simulink library "powerlib_models"  (Simulink 6.0)
settings: Solver=ode45  SolverMode=SingleTasking  StartTime=0.0  StopTime=10.0  RelTol=1e-3
values from neighbouring files (symbols this model uses):
  Ts = get(handles.edit1,'string')    [powergui.m]
undefined symbols (not defined in the file or in its folder): A, a0, a1, a2, a3, a4, a5, Ac, Amplitude, Amplitudes, B, BaseCurrent, BaseFlux, Bc, C, Capacitance, Cc, Columns, ConnectionType, Cs, ctrl, current, Current, damp, Dc, Dd, DiscIntNeverNeededParam, dref, dwo, exc, excAxis, F, Flux, fnom, Frequency, FreqVps, Gain1, gate, GH, GHd, GI, GId, GL, GLd, H, HarmonicGeneration, HT, hyd, I1_init, ib, ib2, Id1o, Inductance, InitialFlux, InitialSlope, io, Iq1o, isfinite, j, J ... (+138)
libraries: powerlib_models x32, powerlib_extras x4
(part 6 of 11)

== system powerlib_models/Continuous/GTO-IGBT Bridge/Vf  ==
  status_GTO : Inport  Port=1  LatchInput=off
  Switch : Switch  Threshold=0.5  InputSameDT=on
  Vf device : Constant  Value=Vf*ones(nb_switch,1)
  Vf diode : Constant  Value=-Vfd*ones(nb_switch,1)
  Vf : Outport  InitialOutput=[0]
  wires:
  status_GTO/1 -> Switch/2
  Switch/1 -> Vf/1
  Vf diode/1 -> Switch/3
  Vf device/1 -> Switch/1

== system powerlib_models/Continuous/HTG/PID ==
  error : Inport  Port=1  LatchInput=off
  Derivative : TransferFcn  Numerator=[ kd 0]  Denominator=[ td 1 ]
  Integral : Gain  Gain=ki  SaturateOnIntegerOverflow=on
  Integrator1 : Integrator  InitialCondition=go
  Proportional : Gain  Gain=kp  SaturateOnIntegerOverflow=on
  Sum : Sum  Inputs=+++  SaturateOnIntegerOverflow=on  InputSameDT=on
  Output : Outport  InitialOutput=0
  wires:
  Integrator1/1 -> Sum/2
  Integral/1 -> Integrator1/1
  error/1 -> Integral/1, Proportional/1, Derivative/1
  Sum/1 -> Output/1
  Derivative/1 -> Sum/3
  Proportional/1 -> Sum/1

== system powerlib_models/Continuous/HTG/servo-motor ==
  regulator's output : Inport  Port=1  LatchInput=off
  Sum4 : Sum  Inputs=+-  SaturateOnIntegerOverflow=on  InputSameDT=on
  position : Integrator  InitialCondition=go  LimitOutput=on  UpperSaturationLimit=gmax  LowerSaturationLimit=gmin
  servo- motor : TransferFcn  Numerator=[ka]  Denominator=[ta 1]
  speed limit : Saturate  UpperLimit=vgmax  LowerLimit=vgmin
  gate opening : Outport  InitialOutput=0
  wires:
  position/1 -> Sum4/2, gate opening/1
  speed limit/1 -> position/1
  servo- motor/1 -> speed limit/1
  Sum4/1 -> servo- motor/1
  regulator's output/1 -> Sum4/1

== system powerlib_models/Continuous/HTG/turbine ==
  dw : Inport  Port=1  LatchInput=off
  gate opening : Inport  Port=2  LatchInput=off
  Constant : Constant  Orientation=left
  Fcn : Fcn  Expr=(u(2)/u(1))^2
  Gain2 : Gain  Orientation=left  Gain=1/tw  SaturateOnIntegerOverflow=on
  Integrator : Integrator  Orientation=left  InitialCondition=po
  Mux : Mux  Inputs=2
  Product : Product  SaturateOnIntegerOverflow=on  InputSameDT=on
  Sum2 : Sum  Inputs=-+  SaturateOnIntegerOverflow=on  InputSameDT=on
  Sum3 : Sum  Orientation=left  Inputs=-+  SaturateOnIntegerOverflow=on  InputSameDT=on
  beta : Gain  Gain=beta  SaturateOnIntegerOverflow=on
  turbine gain : Gain  Gain=1/(gmax-gmin)  SaturateOnIntegerOverflow=on
  Pm : Outport  InitialOutput=0
  wires:
  turbine gain/1 -> Mux/1
  gate opening/1 -> turbine gain/1
  Integrator/1 -> Product/2, Mux/2
  Mux/1 -> Fcn/1
  Fcn/1 -> Sum2/2
  Constant/1 -> Sum3/2
  Product/1 -> Pm/1
  Sum3/1 -> Gain2/1
  Gain2/1 -> Integrator/1
  Sum2/1 -> Sum3/1, Product/1
  beta/1 -> Sum2/1
  dw/1 -> beta/1

== system powerlib_models/Continuous/MBPSS/Transfer function for detailed model (HF) ==
  On : Inport  Port=1  LatchInput=off
  "HFpos " : Inport  Port=2  LatchInput=off
  "HFneg " : Inport  Port=3  LatchInput=off
  Switch1 : Switch  Threshold=0.5  InputSameDT=on
  Switch2 : Switch  Threshold=0.5  InputSameDT=on
  Transfer functions for detailed stabilizer : Subsystem  TreatAsAtomicUnit=on
  Transfer functions for detailed stabilizer2 : Subsystem  TreatAsAtomicUnit=on
  HFpos : Outport
  HFneg : Outport  Port=2
  wires:
  Transfer functions for detailed stabilizer/1(Out1) -> Switch1/1
  "HFpos "/1 -> Transfer functions for detailed stabilizer/1(In1), Switch1/3
  Switch1/1 -> HFpos/1
  "HFneg "/1 -> Transfer functions for detailed stabilizer2/1(In1), Switch2/3
  Switch2/1 -> HFneg/1
  Transfer functions for detailed stabilizer2/1(Out1) -> Switch2/1
  On/1 -> Transfer functions for detailed stabilizer/Enable, Switch1/2, Switch2/2, Transfer functions for detailed stabilizer2/Enable

== system powerlib_models/Continuous/MBPSS/Transfer function for detailed model (IF) ==
  On : Inport  Port=1  LatchInput=off
  "IFpos " : Inport  Port=2  LatchInput=off
  "IFneg " : Inport  Port=3  LatchInput=off
  Switch1 : Switch  Threshold=0.5  InputSameDT=on
  Switch2 : Switch  Threshold=0.5  InputSameDT=on
  Transfer functions for detailed stabilizer : Subsystem  TreatAsAtomicUnit=on
  Transfer functions for detailed stabilizer2 : Subsystem  TreatAsAtomicUnit=on
  IFpos : Outport
  LFneg : Outport  Port=2
  wires:
  On/1 -> Transfer functions for detailed stabilizer2/Enable, Switch2/2, Switch1/2, Transfer functions for detailed stabilizer/Enable
  Transfer functions for detailed stabilizer2/1(Out1) -> Switch2/1
  Switch2/1 -> LFneg/1
  "IFneg "/1 -> Switch2/3, Transfer functions for detailed stabilizer2/1(In1)
  Switch1/1 -> IFpos/1
  "IFpos "/1 -> Switch1/3, Transfer functions for detailed stabilizer/1(In1)
  Transfer functions for detailed stabilizer/1(Out1) -> Switch1/1

== system powerlib_models/Continuous/MBPSS/Transfer function for detailed model (LF) ==
  On : Inport  Port=1  LatchInput=off
  "LFpos " : Inport  Port=2  LatchInput=off
  "LFneg " : Inport  Port=3  LatchInput=off
  Switch1 : Switch  Threshold=0.5  InputSameDT=on
  Switch2 : Switch  Threshold=0.5  InputSameDT=on
  Transfer functions for detailed stabilizer : Subsystem  TreatAsAtomicUnit=on
  Transfer functions for detailed stabilizer2 : Subsystem  TreatAsAtomicUnit=on
  LFpos : Outport
  LFneg : Outport  Port=2
  wires:
  Transfer functions for detailed stabilizer/1(Out1) -> Switch1/1
  "LFpos "/1 -> Transfer functions for detailed stabilizer/1(In1), Switch1/3
  Switch1/1 -> LFpos/1
  "LFneg "/1 -> Transfer functions for detailed stabilizer2/1(In1), Switch2/3
  Switch2/1 -> LFneg/1
  Transfer functions for detailed stabilizer2/1(Out1) -> Switch2/1
  On/1 -> Transfer functions for detailed stabilizer/Enable, Switch1/2, Switch2/2, Transfer functions for detailed stabilizer2/Enable

== system powerlib_models/Continuous/PM_synchronous_machine/abc2qd ==
  note: This subsystem converts Vab and Vbc to Vd,Vq. The sine and cosine com-
      | puted here are sent to the inverse transformation subsystem dq2abc.
  Vab,Vbc : Inport  Port=1  LatchInput=off
  the : Inport  Port=2  LatchInput=off
  Elementary Math : ElementaryMath
  Elementary Math1 : ElementaryMath  Operator=cos
  Fcn2 : Fcn  Expr=(u[4]*(2*u[1]+u[2]) + (sqrt3*u[2]*u[3])) * one_third
  Fcn3 : Fcn  Expr=(u[3]*(2*u[1]+u[2]) + (-sqrt3*u[2]*u[4])) * one_third
  Mux1 : Mux  Inputs=[ 2 2 ]
  Mux2 : Mux  Inputs=2
  Mux3 : Mux  Inputs=2
  s,c : Outport  InitialOutput=0
  vq,vd : Outport  Port=2  InitialOutput=0
  wires:
  the/1 -> Elementary Math1/1, Elementary Math/1
  Elementary Math1/1 -> Mux3/2
  Elementary Math/1 -> Mux3/1
  Vab,Vbc/1 -> Mux1/1
  Mux2/1 -> vq,vd/1
  Fcn3/1 -> Mux2/2
  Fcn2/1 -> Mux2/1
  Mux3/1 -> Mux1/2, s,c/1
  Mux1/1 -> Fcn3/1, Fcn2/1

== system powerlib_models/Continuous/PM_synchronous_machine/iq,id ==
  vq,vd : Inport  Port=1  LatchInput=off
  we : Inport  Port=2  LatchInput=off
  Demux : Demux  Outputs=2
  Mux : Mux  Inputs=2
  id : Subsystem
  iq : Subsystem
  iq,id : Outport  InitialOutput=0
  wires:
  Mux/1 -> iq,id/1
  vq,vd/1 -> Demux/1
  Demux/1 -> iq/1(vq)
  Demux/2 -> id/3(vd)
  iq/1(iq) -> id/1(iq), Mux/1
  we/1 -> id/2(we), iq/2(we)
  id/1(id) -> iq/3(id), Mux/2

== system powerlib_models/Continuous/PM_synchronous_machine/qd2abc ==
  s,c : Inport  Port=1  LatchInput=off
  iq,id : Inport  Port=2  LatchInput=off
  Fcn : Fcn  Expr=u[3]*u[2] + u[4]*u[1]
  Fcn1 : Fcn  Expr=(u[2]*(-u[3]-sqrt3*u[4]) + u[1]*(sqrt3*u[3]-u[4]))*0.5
  Mux : Mux  Inputs=[2,2]
  Mux2 : Mux  Inputs=3
  Sum : Sum  Orientation=down  Inputs=--  SaturateOnIntegerOverflow=on  InputSameDT=on
  is : Outport  InitialOutput=0
  wires:
  Mux2/1 -> is/1
  Fcn1/1 -> Sum/1, Mux2/2
  Fcn/1 -> Sum/2, Mux2/1
  Sum/1 -> Mux2/3
  iq,id/1 -> Mux/2
  s,c/1 -> Mux/1
  Mux/1 -> Fcn1/1, Fcn/1

== system powerlib_models/Continuous/PSS/Sensor ==
  In : Inport  Port=1  LatchInput=off
  State-Space : StateSpace  A=Ac  B=Bc  C=Cc  D=Dc  X0=x0c
  Out : Outport  InitialOutput=0
  wires:
  In/1 -> State-Space/1
  State-Space/1 -> Out/1

== system powerlib_models/Continuous/PSS/Wash-out ==
  In : Inport  Port=1  LatchInput=off
  State-Space : StateSpace  A=Ac  B=Bc  C=Cc  D=Dc  X0=x0c
  Out : Outport  InitialOutput=0
  wires:
  In/1 -> State-Space/1
  State-Space/1 -> Out/1

== system powerlib_models/Continuous/Three-Level Bridge/2-level GTO-IGBT Bridge  Logic (modified) ==
  note: Diode Logic :
      | 1) Diodes are blocked when complementary GTOs are switched on
  note: Note 3: See Sw3 logic
  v : Inport  Port=1  LatchInput=off
  g : Inport  Port=2  LatchInput=off
  Block12 : Inport  Port=3  LatchInput=off
  Trig12 : Inport  Port=4  LatchInput=off
  Data Type  Conversion2 : DataTypeConversion  OutDataTypeMode=double  SaturateOnIntegerOverflow=on  RndMeth=Zero
  Data Type  Conversion4 : DataTypeConversion  OutDataTypeMode=boolean  SaturateOnIntegerOverflow=on  RndMeth=Zero
  Demux1 : Demux  Outputs=[nb_arm nb_arm]
  Diode Logic : Subsystem
  GTO Logic : Subsystem
  G_D : Logic  Operator=OR
  G_D2 : Logic  Operator=NOT
  G_D3 : Logic  Operator=OR
  G_D4 : Logic  Operator=OR
  Gain : Gain  Orientation=up  Gain=-1  SaturateOnIntegerOverflow=on
  Gain1 : Gain  Gain=2  SaturateOnIntegerOverflow=on
  Memory : Memory
  Memory1 : Memory
  Note 3 : Logic
  Select_Block3 : Selector  Elements=Block3Elements  InputPortWidth=nb_switch
  Select_Vsw : Selector  Elements=VswElements  InputPortWidth=nb_arm*3
  "Vf " : Subsystem
  status : Outport
  Vf : Outport  Port=2
  Block3 : Outport  Port=3
  status_GTO : Outport  Port=4
  wires:
  Demux1/2 -> G_D3/2
  Demux1/1 -> G_D3/1
  Select_Block3/1 -> Demux1/1
  Select_Vsw/1 -> GTO Logic/1(Vak), Gain/1
  Trig12/1 -> G_D4/2
  Note 3/1 -> G_D4/1
  G_D4/1 -> G_D/1
  Memory/1 -> Vf/1
  Data Type  Conversion2/1 -> Memory1/1
  G_D/1 -> Data Type  Conversion2/1
  Memory1/1 -> status/1
  Data Type  Conversion4/1 -> GTO Logic/2(G)
  g/1 -> Data Type  Conversion4/1
  GTO Logic/1(status) -> status_GTO/1, "Vf "/1(status_GTO), Diode Logic/2(G), G_D/2
  "Vf "/1(Vf) -> Gain1/1
  v/1 -> Select_Vsw/1
  Gain/1 -> Diode Logic/1(Vak)
  Diode Logic/2(block) -> Select_Block3/1
  Diode Logic/1(status) -> Note 3/1
  Block12/1 -> G_D2/1
  G_D2/1 -> Note 3/2
  Gain1/1 -> Memory/1
  G_D3/1 -> Block3/1

== system powerlib_models/Continuous/Three-Level Bridge/Input ==
  note: This block is required when the "pulses" input is not connected
  In : Inport  Port=1  LatchInput=off
  Constant : Constant
  require : Logic  OutDataTypeMode=Specify via dialog  LogicDataType=float('double')
  Out : Outport
  wires:
  require/1 -> Out/1
  In/1 -> require/1
  Constant/1 -> require/2

== system powerlib_models/Continuous/Three-Level Bridge/SubSystem ==
  note: (or B or C)
  note: (or B or C)
  note: <======>
  note: |
      | |
      | |
      | |
      | |
      | [Sw2]
      | |
      | |
      | |
      | |
  note: |
      | |
      | |
      | |
      | |
      | [Sw1]
      | |
      | |
      | |
      | |
  note: + Vdc ------------
  note: ---------- A
  note: + Vdc --------------------------
  note: - Vdc--------------------------
  note: N ----------
  note: |
      | |
      | |
      | |
      | |
      | |
      | |
      | |
      | |
      | |
      | |
  note: ------------ A
  note: -----<-[D6]---------
  note: -------[D5]-->-------
  note: |
      | |
      | [Q4 - D4]
      | |
      | |
      | |
  note: |
      | |
      | [Q3 - D3]
      | |
      | |
  note: |
      | |
      | [Q2 - D2]
      | |
      | |
  note: |
      | |
      | |
      | [Q1 - D1]
      | |
      | |
  note: -[Sw3]-----
  note: N ----
  note: - Vdc ------------
  note: D5, D6 : Clamping diodes

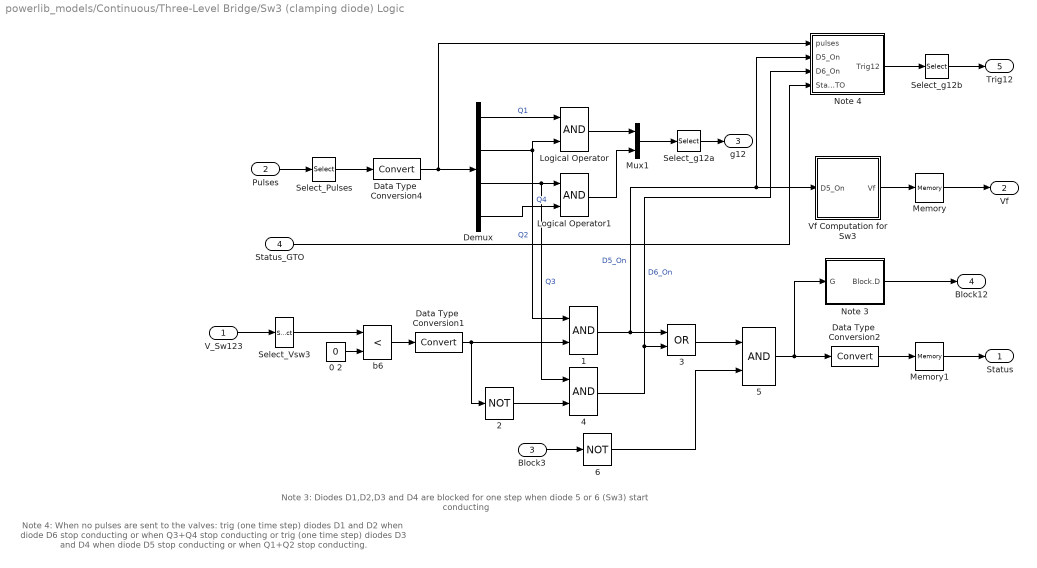
== system powerlib_models/Continuous/Three-Level Bridge/Sw3 (clamping diode) Logic ==
  note: Note 4: When no pulses are sent to the valves:
      | trig (one time step) diodes D1 and D2 when diode D6 stop conducting or when Q3+Q4 stop conducting
      | or trig (one time step) diodes D3 and D4 when diode D5 stop conducting or when Q1+Q2 stop conducting.
  note: Note 3: Diodes D1,D2,D3 and D4 are blocked for one step when diode 5 or 6 (Sw3) start conducting
  V_Sw123 : Inport  Port=1  LatchInput=off
  Pulses : Inport  Port=2  LatchInput=off
  Block3 : Inport  Port=3  LatchInput=off
  Status_GTO : Inport  Port=4  LatchInput=off
  0 2 : Constant  Value=0
  1 : Logic
  2 : Logic  Operator=NOT
  3 : Logic  Operator=OR
  4 : Logic
  5 : Logic
  6 : Logic  Operator=NOT
  Data Type  Conversion1 : DataTypeConversion  OutDataTypeMode=boolean  SaturateOnIntegerOverflow=on  RndMeth=Zero
  Data Type  Conversion2 : DataTypeConversion  OutDataTypeMode=double  SaturateOnIntegerOverflow=on  RndMeth=Zero
  Data Type  Conversion4 : DataTypeConversion  OutDataTypeMode=boolean  SaturateOnIntegerOverflow=on  RndMeth=Zero
  Demux : Demux  Outputs=[nb_arm nb_arm nb_arm nb_arm]
  Logical Operator : Logic
  Logical Operator1 : Logic
  Memory : Memory
  Memory1 : Memory
  Mux1 : Mux  Inputs=[nb_arm nb_arm]
  Note 3 : Subsystem
  Note 4 : Subsystem
  Select_Pulses : Selector  Elements=PulseElements  InputPortWidth=nb_arm*4
  Select_Vsw3 : Selector  Elements=Vsw3Elements  InputPortWidth=nb_arm*3
  Select_g12a : Selector  Elements=g12Elements  InputPortWidth=nb_arm*2
  Select_g12b : Selector  Elements=g12Elements  InputPortWidth=nb_arm*2
  Vf Computation for Sw3 : Subsystem
  b6 : RelationalOperator  Operator=<  InputSameDT=on
  Status : Outport
  Vf : Outport  Port=2
  g12 : Outport  Port=3
  Block12 : Outport  Port=4
  Trig12 : Outport  Port=5
  wires:
  Status_GTO/1 -> Note 4/4(Status_GTO)
  Select_Pulses/1 -> Data Type  Conversion4/1
  Note 4/1(Trig12) -> Select_g12b/1
  Data Type  Conversion2/1 -> Memory1/1
  6/1 -> 5/2
  3/1 -> 5/1
  1/1 -> Note 4/2(D5_On), Vf Computation for Sw3/1(D5_On), 3/1  "D5_On"
  4/1 -> Note 4/3(D6_On), 3/2  "D6_On"
  Data Type  Conversion1/1 -> 2/1, 1/2
  b6/1 -> Data Type  Conversion1/1
  Logical Operator1/1 -> Mux1/2
  Demux/4 -> Logical Operator1/2  "Q4"
  Demux/3 -> Logical Operator1/1, 4/1  "Q3"
  Demux/2 -> 1/1, Logical Operator/2  "Q2"
  Demux/1 -> Logical Operator/1  "Q1"
  Data Type  Conversion4/1 -> Note 4/1(pulses), Demux/1
  Memory/1 -> Vf/1
  Vf Computation for Sw3/1(Vf) -> Memory/1
  Mux1/1 -> Select_g12a/1
  Pulses/1 -> Select_Pulses/1
  0 2/1 -> b6/2
  V_Sw123/1 -> Select_Vsw3/1
  2/1 -> 4/2
  Memory1/1 -> Status/1
  Block3/1 -> 6/1
  Note 3/1(Block.D) -> Block12/1
  5/1 -> Data Type  Conversion2/1, Note 3/1(G)
  Select_Vsw3/1 -> b6/1
  Logical Operator/1 -> Mux1/1
  Select_g12a/1 -> g12/1
  Select_g12b/1 -> Trig12/1

== system powerlib_models/Continuous/asynchronous_machine/Mutual fluxes ==
  phiqr,phidr : Inport  Port=1  LatchInput=off
  phiqs,phids : Inport  Port=2  LatchInput=off
  1\Llr : Gain  Gain=1/Llr  SaturateOnIntegerOverflow=on
  1\Llr1 : Gain  Gain=Laq  SaturateOnIntegerOverflow=on
  1\Llr2 : Gain  Gain=Lad  SaturateOnIntegerOverflow=on
  1\Lls : Gain  Gain=1/Lls  SaturateOnIntegerOverflow=on
  Demux1 : Demux  Outputs=2
  Demux2 : Demux  Outputs=2
  Mux3 : Mux  Inputs=2
  Sum : Sum  Inputs=|++  SaturateOnIntegerOverflow=on  InputSameDT=on
  Sum1 : Sum  Inputs=++|  SaturateOnIntegerOverflow=on  InputSameDT=on
  phimq,phimd : Outport
  wires:
  Sum1/1 -> 1\Llr2/1
  phiqs,phids/1 -> 1\Lls/1
  phiqr,phidr/1 -> 1\Llr/1
  1\Llr/1 -> Demux1/1
  Demux1/1 -> Sum/1
  Sum/1 -> 1\Llr1/1
  1\Lls/1 -> Demux2/1
  Demux2/1 -> Sum/2
  Demux2/2 -> Sum1/2
  Demux1/2 -> Sum1/1
  1\Llr1/1 -> Mux3/1
  1\Llr2/1 -> Mux3/2
  Mux3/1 -> phimq,phimd/1

== system powerlib_models/Continuous/asynchronous_machine/Rotor ==
  vqr,vdr : Inport  Port=1  LatchInput=off
  w-wr : Inport  Port=2  LatchInput=off
  phimq,phimd : Inport  Port=3  LatchInput=off
  1\Llr : Gain  Gain=1/Llr  SaturateOnIntegerOverflow=on
  1\Llr1 : Gain  Gain=Rr  SaturateOnIntegerOverflow=on
  1\Llr2 : Gain  Gain=1/Llr  SaturateOnIntegerOverflow=on
  1\Llr3 : Gain  Gain=Rr  SaturateOnIntegerOverflow=on
  Demux : Demux  Outputs=2
  Demux1 : Demux  Outputs=2
  Mux2 : Mux  Inputs=2
  Mux3 : Mux  Inputs=2
  Product : Product  SaturateOnIntegerOverflow=on  InputSameDT=on
  Product1 : Product  Orientation=left  SaturateOnIntegerOverflow=on  InputSameDT=on
  Sum1 : Sum  Inputs=++-||  SaturateOnIntegerOverflow=on  InputSameDT=on
  Sum2 : Sum  Inputs=+--  SaturateOnIntegerOverflow=on  InputSameDT=on
  Sum3 : Sum  Inputs=+-|  SaturateOnIntegerOverflow=on  InputSameDT=on
  Sum4 : Sum  Inputs=-+|  SaturateOnIntegerOverflow=on  InputSameDT=on
  phidr : Integrator  InitialCondition=phirdo
  phiqr : Integrator  InitialCondition=phirqo
  web1 : Gain  Gain=web_psb  SaturateOnIntegerOverflow=on
  web_psb : Gain  Gain=web_psb  SaturateOnIntegerOverflow=on
  iqr,idr : Outport
  phiqr,phidr : Outport  Port=2
  wires:
  phimq,phimd/1 -> Demux1/1
  Demux1/1 -> Sum3/2
  Demux/1 -> Sum2/1
  Sum3/1 -> 1\Llr/1
  1\Llr1/1 -> Sum2/3
  1\Llr/1 -> 1\Llr1/1, Mux2/1  "iqr"
  Mux2/1 -> iqr,idr/1
  Demux1/2 -> Sum4/1
  Sum4/1 -> 1\Llr2/1
  1\Llr2/1 -> Mux2/2, 1\Llr3/1  "idr"
  1\Llr3/1 -> Sum1/3
  Demux/2 -> Sum1/2
  Product1/1 -> Sum1/1
  vqr,vdr/1 -> Demux/1
  phidr/1 -> Mux3/2, Product/1, Sum4/2
  Sum2/1 -> web_psb/1
  web_psb/1 -> phiqr/1
  Product/1 -> Sum2/2
  w-wr/1 -> Product1/1, Product/2
  Sum1/1 -> web1/1
  web1/1 -> phidr/1
  phiqr/1 -> Sum3/1, Product1/2, Mux3/1  "phiqr"
  Mux3/1 -> phiqr,phidr/1

== system powerlib_models/Continuous/asynchronous_machine/Stator ==
  phimq,phimd : Inport  Port=1  LatchInput=off
  vqs,vds : Inport  Port=2  LatchInput=off
  w : Inport  Port=3  LatchInput=off
  1\Llr : Gain  Gain=1/Lls  SaturateOnIntegerOverflow=on
  1\Llr1 : Gain  Gain=Rs  SaturateOnIntegerOverflow=on
  1\Llr2 : Gain  Gain=1/Lls  SaturateOnIntegerOverflow=on
  1\Llr3 : Gain  Gain=Rs  SaturateOnIntegerOverflow=on
  Demux : Demux  Outputs=2
  Demux1 : Demux  Outputs=2
  Mux2 : Mux  Inputs=2
  Mux3 : Mux  Inputs=2
  Mux4 : Mux  Inputs=2
  Product : Product  SaturateOnIntegerOverflow=on  InputSameDT=on
  Product1 : Product  SaturateOnIntegerOverflow=on  InputSameDT=on
  Sum1 : Sum  Inputs=++-||  SaturateOnIntegerOverflow=on  InputSameDT=on
  Sum2 : Sum  Inputs=--+  SaturateOnIntegerOverflow=on  InputSameDT=on
  Sum3 : Sum  Inputs=-+  SaturateOnIntegerOverflow=on  InputSameDT=on
  Sum4 : Sum  Inputs=+-|  SaturateOnIntegerOverflow=on  InputSameDT=on
  phids : Integrator  InitialCondition=phisdo
  phiqs : Integrator  InitialCondition=phisqo
  web1 : Gain  Gain=web_psb  SaturateOnIntegerOverflow=on
  web_psb : Gain  Gain=web_psb  SaturateOnIntegerOverflow=on
  phiqs,phids : Outport
  iqs,ids : Outport  Port=2
  phis,is : Outport  Port=3
  wires:
  Mux4/1 -> phis,is/1
  Mux3/1 -> Mux4/1, phiqs,phids/1
  Product1/1 -> Sum1/1
  Demux/2 -> Sum1/2
  phids/1 -> Mux3/2, Sum3/2, Product/2
  Sum1/1 -> web1/1
  web1/1 -> phids/1
  1\Llr3/1 -> Sum1/3
  1\Llr2/1 -> Mux2/2, 1\Llr3/1  "ids"
  Sum3/1 -> 1\Llr2/1
  Demux1/2 -> Sum3/1
  w/1 -> Product1/1, Product/1
  Mux2/1 -> Mux4/2, iqs,ids/1
  phiqs/1 -> Sum4/1, Product1/2, Mux3/1
  web_psb/1 -> phiqs/1
  Product/1 -> Sum2/2
  Demux/1 -> Sum2/3
  Sum2/1 -> web_psb/1
  vqs,vds/1 -> Demux/1
  1\Llr1/1 -> Sum2/1
  1\Llr/1 -> 1\Llr1/1, Mux2/1  "iqs"
  Sum4/1 -> 1\Llr/1
  Demux1/1 -> Sum4/2
  phimq,phimd/1 -> Demux1/1

== system powerlib_models/Continuous/asynchronous_machine/abc2qd ==
  v : Inport  Port=1  LatchInput=off
  sin,cos : Inport  Port=2  LatchInput=off
  1_Vb : Gain  Gain=1/Vb  SaturateOnIntegerOverflow=on
  Constant : Constant  Orientation=down  Value=ctrl==1
  Constant1 : Constant  Orientation=down  Value=ctrl==2
  Constant2 : Constant  Orientation=down  Value=ctrl==3
  Constant3 : Constant  Orientation=down  Value=ctrl
  Constant4 : Constant  Orientation=left  Value=ctrl
  Multiport Switch : MultiPortSwitch  Inputs=3  InputSameDT=on
  Multiport Switch1 : MultiPortSwitch  Inputs=3  InputSameDT=on
  Mux : Mux  Inputs=2
  Rotor reference frame : Subsystem  TreatAsAtomicUnit=on
      mask Display: disp('Rotor\nreference\nframe')
  Stationary reference frame : Subsystem  TreatAsAtomicUnit=on
      mask Display: disp('Stationary\nreference\nframe')
  Synchronous reference frame : Subsystem  TreatAsAtomicUnit=on
      mask Display: disp('Synchronous\nreference\nframe')
  transit : Subsystem
  vqr,vdr : Outport
  vqs,vds : Outport  Port=2
  wires:
  v/1 -> transit/1(vu)
  Constant/1 -> Rotor reference frame/Enable
  Constant1/1 -> Stationary reference frame/Enable
  Constant2/1 -> Synchronous reference frame/Enable
  Multiport Switch1/1 -> vqs,vds/1
  Rotor reference frame/1(vqr,vdr) -> Multiport Switch/2
  Stationary reference frame/1(vqr,vdr) -> Multiport Switch/3
  Synchronous reference frame/1(vqr,vdr) -> Multiport Switch/4
  Rotor reference frame/2(vqs,vds) -> Multiport Switch1/2
  Stationary reference frame/2(vqs,vds) -> Multiport Switch1/3
  Synchronous reference frame/2(vqs,vds) -> Multiport Switch1/4
  Multiport Switch/1 -> vqr,vdr/1
  sin,cos/1 -> Mux/2
  Mux/1 -> Rotor reference frame/1(In1), Stationary reference frame/1(In1), Synchronous reference frame/1(In1)
  1_Vb/1 -> Mux/1
  Constant3/1 -> Multiport Switch/1
  Constant4/1 -> Multiport Switch1/1
  transit/1(vr,vs) -> 1_Vb/1

== system powerlib_models/Continuous/asynchronous_machine/dq2abc ==
  sin,cos : Inport  Port=1  LatchInput=off
  iqr,idr : Inport  Port=2  LatchInput=off
  iqs,ids : Inport  Port=3  LatchInput=off
  Constant : Constant  Orientation=down  Value=ctrl==1
  Constant1 : Constant  Orientation=down  Value=ctrl==2
  Constant2 : Constant  Orientation=down  Value=ctrl==3
  Constant3 : Constant  Orientation=down  Value=ctrl
  Constant4 : Constant  Orientation=left  Value=ctrl
  Multiport Switch : MultiPortSwitch  Inputs=3  InputSameDT=on
  Multiport Switch1 : MultiPortSwitch  Inputs=3  InputSameDT=on
  Mux : Mux  Inputs=3
  Mux1 : Mux  Inputs=2
  Mux2 : Mux  Inputs=2
  Mux3 : Mux  Inputs=2
  Rotor reference frame : Subsystem  TreatAsAtomicUnit=on
      mask Display: disp('Rotor\nreference\nframe')
  Selector : Selector  Elements=elements2  InputPortWidth=4
  Stationary reference frame : Subsystem  TreatAsAtomicUnit=on
      mask Display: disp('Stationary\nreference\nframe')
  Sum2 : Sum  Inputs=-  SaturateOnIntegerOverflow=on  InputSameDT=on
  Sum3 : Sum  Inputs=-  SaturateOnIntegerOverflow=on  InputSameDT=on
  Synchronous reference frame : Subsystem  TreatAsAtomicUnit=on
      mask Display: disp('Synchronous\nreference\nframe')
  ib : Gain  Gain=ib  SaturateOnIntegerOverflow=on
  irab,isab : Outport
  irabc : Outport  Port=2
  isabc : Outport  Port=3
  wires:
  Constant/1 -> Rotor reference frame/Enable
  Constant1/1 -> Stationary reference frame/Enable
  Constant2/1 -> Synchronous reference frame/Enable
  Rotor reference frame/1(ira,irb) -> Multiport Switch/2
  Stationary reference frame/1(ira,irb) -> Multiport Switch/3
  Synchronous reference frame/1(ira,irb) -> Multiport Switch/4
  Stationary reference frame/2(isa,isb) -> Multiport Switch1/3
  Synchronous reference frame/2(isa,isb) -> Multiport Switch1/4
  Mux/1 -> Rotor reference frame/1(In1), Stationary reference frame/1(In1), Synchronous reference frame/1(In1)
  iqs,ids/1 -> Mux/2
  iqr,idr/1 -> Mux/1
  Multiport Switch/1 -> Mux2/1, Mux1/1, Sum2/1
  Mux2/1 -> irabc/1
  Multiport Switch1/1 -> Mux1/2, Sum3/1, Mux3/1
  Sum2/1 -> Mux2/2
  sin,cos/1 -> Mux/3
  Rotor reference frame/2(isa,isb) -> Multiport Switch1/2
  Mux1/1 -> ib/1
  Constant3/1 -> Multiport Switch/1
  Constant4/1 -> Multiport Switch1/1
  Sum3/1 -> Mux3/2
  Mux3/1 -> isabc/1
  ib/1 -> Selector/1
  Selector/1 -> irab,isab/1

== system powerlib_models/Continuous/asynchronous_machine/sin,cos ==
  thr,wr : Inport  Port=1  LatchInput=off
  Constant : Constant  Orientation=down  Value=ctrl<3
  Constant1 : Constant  Value=ctrl
  Constant2 : Constant  Value=0
  Constant3 : Constant  Orientation=down  Value=ctrl==3
  Constant4 : Constant  Value=ctrl
  Constant5 : Constant  Value=0
  Constant6 : Constant
  Gain : Gain  Gain=-1  SaturateOnIntegerOverflow=on
  Multiport Switch : MultiPortSwitch  Inputs=3  InputSameDT=on
  Multiport Switch1 : MultiPortSwitch  Inputs=3  InputSameDT=on
  Selector : Selector  InputPortWidth=2
  Selector1 : Selector  Elements=2  InputPortWidth=2
  Switch : Switch  Threshold=0.5  InputSameDT=on
  sin(beta),cos(beta),sin(th),cos(th) : Subsystem  TreatAsAtomicUnit=on
  sin(thr),cos(thr) : Subsystem  TreatAsAtomicUnit=on
  sin,cos : Outport
  w-wr : Outport  Port=2
  w : Outport  Port=3
  wires:
  Multiport Switch1/1 -> w/1
  Constant6/1 -> Multiport Switch1/4
  Constant5/1 -> Multiport Switch1/3
  Constant4/1 -> Multiport Switch1/1
  Selector1/1 -> Multiport Switch1/2, Gain/1
  Gain/1 -> Multiport Switch/3  "-wr"
  sin(beta),cos(beta),sin(th),cos(th)/1("sin(beta),cos(beta), sin(th),cos(th)") -> Switch/3
  sin(thr),cos(thr)/1(sin(thr),cos(thr)) -> Switch/1
  Multiport Switch/1 -> w-wr/1
  Constant2/1 -> Multiport Switch/2
  Constant1/1 -> Multiport Switch/1
  sin(beta),cos(beta),sin(th),cos(th)/2(we-wr) -> Multiport Switch/4
  Constant3/1 -> sin(beta),cos(beta),sin(th),cos(th)/Enable
  Switch/1 -> sin,cos/1
  Selector/1 -> sin(thr),cos(thr)/1(thr)
  thr,wr/1 -> Selector1/1, sin(beta),cos(beta),sin(th),cos(th)/1(thr,wr), Selector/1
  Constant/1 -> Switch/2, sin(thr),cos(thr)/Enable

== system powerlib_models/Continuous/breaker/Break Algebraic Loop ==
  In1 : Inport  Port=1  LatchInput=off
  0 2 : Constant  Value=0.001
  Data Type  Conversion : DataTypeConversion  OutDataTypeMode=double  SaturateOnIntegerOverflow=on  RndMeth=Zero
  Data Type  Conversion1 : DataTypeConversion  OutDataTypeMode=double  SaturateOnIntegerOverflow=on  RndMeth=Zero
  Integrator : Integrator  InitialCondition=0.00101*(istate&1)  LimitOutput=on  UpperSaturationLimit=0.00101
  R_device : Gain  Gain=1e7  SaturateOnIntegerOverflow=on
  Relational Operator1 : RelationalOperator  Operator=>  InputSameDT=on
  Vak-Vf-Ron*Iak : Sum  Inputs=+-  SaturateOnIntegerOverflow=on  InputSameDT=on
  Out1 : Outport
  wires:
  Data Type  Conversion/1 -> Out1/1
  In1/1 -> Data Type  Conversion1/1
  Data Type  Conversion1/1 -> Vak-Vf-Ron*Iak/1
  R_device/1 -> Integrator/1
  Vak-Vf-Ron*Iak/1 -> R_device/1
  Integrator/1 -> Vak-Vf-Ron*Iak/2, Relational Operator1/1
  0 2/1 -> Relational Operator1/2
  Relational Operator1/1 -> Data Type  Conversion/1

== system powerlib_models/Continuous/detailed_thyristor (logical)/Break Alg. Loop ==
  In1 : Inport  Port=1  LatchInput=off
  0 2 : Constant  Value=0.001
  Data Type  Conversion : DataTypeConversion  OutDataTypeMode=double  SaturateOnIntegerOverflow=on  RndMeth=Zero
  Data Type  Conversion1 : DataTypeConversion  OutDataTypeMode=double  SaturateOnIntegerOverflow=on  RndMeth=Zero
  Integrator : Integrator  LimitOutput=on  UpperSaturationLimit=0.00101
  R_device : Gain  Gain=1e7  SaturateOnIntegerOverflow=on
  Relational Operator1 : RelationalOperator  Operator=>  InputSameDT=on
  Vak-Vf-Ron*Iak : Sum  Inputs=+-  SaturateOnIntegerOverflow=on  InputSameDT=on
  Out1 : Outport
  wires:
  Relational Operator1/1 -> Data Type  Conversion/1
  0 2/1 -> Relational Operator1/2
  Integrator/1 -> Relational Operator1/1, Vak-Vf-Ron*Iak/2
  Vak-Vf-Ron*Iak/1 -> R_device/1
  R_device/1 -> Integrator/1
  Data Type  Conversion1/1 -> Vak-Vf-Ron*Iak/1
  In1/1 -> Data Type  Conversion1/1
  Data Type  Conversion/1 -> Out1/1

== system powerlib_models/Continuous/diode (logical)/Break Alg. Loop ==
  In1 : Inport  Port=1  LatchInput=off
  0 2 : Constant  Value=0.001
  Data Type  Conversion : DataTypeConversion  OutDataTypeMode=double  SaturateOnIntegerOverflow=on  RndMeth=Zero
  Data Type  Conversion1 : DataTypeConversion  OutDataTypeMode=double  SaturateOnIntegerOverflow=on  RndMeth=Zero
  Integrator : Integrator  LimitOutput=on  UpperSaturationLimit=0.00101
  R_device : Gain  Gain=1e7  SaturateOnIntegerOverflow=on
  Relational Operator1 : RelationalOperator  Operator=>  InputSameDT=on
  Vak-Vf-Ron*Iak : Sum  Inputs=+-  SaturateOnIntegerOverflow=on  InputSameDT=on
  Out1 : Outport
  wires:
  Relational Operator1/1 -> Data Type  Conversion/1
  0 2/1 -> Relational Operator1/2
  Integrator/1 -> Relational Operator1/1, Vak-Vf-Ron*Iak/2
  Vak-Vf-Ron*Iak/1 -> R_device/1
  R_device/1 -> Integrator/1
  Data Type  Conversion1/1 -> Vak-Vf-Ron*Iak/1
  In1/1 -> Data Type  Conversion1/1
  Data Type  Conversion/1 -> Out1/1

== system powerlib_models/Continuous/hysteresis_transformer/Hysteresis ( always SI ) ==
  In1 : Inport  Port=1  LatchInput=off
  Hysteresis main loop + Saturation (Lower Part) : Lookup  DialogController=Simulink.DDGSource  InputValues=LowerFlux  OutputValues=Current  SaturateOnIntegerOverflow=on
  Hysteresis main loop + Saturation. (Upper Part) : Lookup  DialogController=Simulink.DDGSource  InputValues=UpperFlux  OutputValues=Current  SaturateOnIntegerOverflow=on
  Memory : Memory
  SI conversion : Gain  Gain=CurrentBase  SaturateOnIntegerOverflow=on
  Selector : Selector  Elements=2  InputPortWidth=2
  Selector1 : Selector  InputPortWidth=2
  Sfunction : S-Function  FunctionName=sfun_hysteresis  Parameters=sfun_InitialFlux,HT,TransfoNumber,-1,Tolerances,InitialSlope
  Sign : Signum
  Sum : Sum  Inputs=|+-  SaturateOnIntegerOverflow=on  InputSameDT=on
  Switch1 : Switch  InputSameDT=on
  Switch2 : Switch  Threshold=1.5  InputSameDT=on
  pu conversion : Gain  Gain=1/FluxBase  SaturateOnIntegerOverflow=on
  Out1 : Outport
  wires:
  Sum/1 -> Sign/1
  SI conversion/1 -> Switch2/1  "internal loops"
  Selector1/1 -> SI conversion/1
  Selector/1 -> Switch2/2  "Tr"
  Switch1/1 -> Switch2/3
  Switch2/1 -> Out1/1
  Sfunction/1 -> Selector1/1, Selector/1
  pu conversion/1 -> Sfunction/1
  Sign/1 -> Switch1/2
  Memory/1 -> Sum/2
  Hysteresis main loop + Saturation. (Upper Part)/1 -> Switch1/3
  In1/1 -> Sum/1, Memory/1, Hysteresis main loop + Saturation. (Upper Part)/1, Hysteresis main loop + Saturation (Lower Part)/1, pu conversion/1
  Hysteresis main loop + Saturation (Lower Part)/1 -> Switch1/1

== system powerlib_models/Continuous/simplified_sync_mach/Subsystem ==
  i : Inport  Port=1  LatchInput=off
  v : Inport  Port=2  LatchInput=off
  e : Inport  Port=3  LatchInput=off
  theta : Inport  Port=4  LatchInput=off
  wm : Inport  Port=5  LatchInput=off
  Pe : Inport  Port=6  LatchInput=off
  Gain : Gain  Gain=[ ib2*ones(3,1); Vb3*ones(6,1); 1; Nb; Pb ]  SaturateOnIntegerOverflow=on
  Mux : Mux  Inputs=[ 3 3 3 1 1 1 ]
  * : Outport  InitialOutput=0
  wires:
  Gain/1 -> */1
  Mux/1 -> Gain/1
  Pe/1 -> Mux/6
  wm/1 -> Mux/5
  theta/1 -> Mux/4
  e/1 -> Mux/3
  v/1 -> Mux/2
  i/1 -> Mux/1

== system powerlib_models/Continuous/simplified_sync_mach/Vt ==
  note: This subsystem either converts 2 line-to-line voltages to 3 line-to-neutral voltages (internal neutral)
      | and computes floating neutral voltage or directly passes Van,Vbn,Vcn if 4-wire connection.
  V : Inport  Port=1  LatchInput=off
  1_Vb : Gain  Gain=1/Vb  SaturateOnIntegerOverflow=on
  Constant : Constant  Orientation=left  Value=ConnectionType
  Constant1 : Constant  Value=0
  Constant2 : Constant  Value=0
  Data Type  Conversion1 : DataTypeConversion  Orientation=left  OutDataTypeMode=boolean  SaturateOnIntegerOverflow=on  RndMeth=Zero
  Data Type  Conversion2 : DataTypeConversion  OutDataTypeMode=double  SaturateOnIntegerOverflow=on  RndMeth=Zero
  Fcn : Fcn  Expr=u[1]
  Fcn1 : Fcn  Expr=u[2]
  Fcn2 : Fcn  Expr=u[3]
  Gain : Gain  Gain=1/3  SaturateOnIntegerOverflow=on
  LL2LN : Subsystem  TreatAsAtomicUnit=on
  Logical Operator : Logic  Operator=NOT
  Mux : Mux  Inputs=2
  Mux1 : Mux  Inputs=3
  Product : Product  SaturateOnIntegerOverflow=on  InputSameDT=on
  Sum : Sum  Inputs=+  SaturateOnIntegerOverflow=on  InputSameDT=on
  Sum1 : Sum  Inputs=|++  SaturateOnIntegerOverflow=on  InputSameDT=on
  Switch2 : Switch  Threshold=0.5  InputSameDT=on
  Vn : Outport  InitialOutput=0
  Vabc : Outport  Port=2  InitialOutput=0
  wires:
  Data Type  Conversion2/1 -> Product/1
  Logical Operator/1 -> Data Type  Conversion2/1
  Data Type  Conversion1/1 -> Logical Operator/1
  Constant/1 -> Data Type  Conversion1/1, LL2LN/Enable, Switch2/2
  Sum/1 -> Gain/1
  Gain/1 -> Switch2/1
  Constant2/1 -> Switch2/3
  Switch2/1 -> Vn/1
  LL2LN/1(Out1) -> Sum/1, Sum1/1
  Sum1/1 -> Vabc/1
  Constant1/1 -> Mux/2
  Mux/1 -> Fcn/1, Fcn1/1, Fcn2/1
  Fcn/1 -> Mux1/1
  Fcn1/1 -> Mux1/2
  Fcn2/1 -> Mux1/3
  Mux1/1 -> Product/2
  Product/1 -> Sum1/2
  V/1 -> 1_Vb/1
  1_Vb/1 -> LL2LN/1(In1), Mux/1

== system powerlib_models/Continuous/simplified_sync_mach/Z ==
  note: This subsystem models the internal impedance of
      | the machine, which consists of  a series RL circuit.
  e : Inport  Port=1  LatchInput=off
  v : Inport  Port=2  LatchInput=off
  1/L : Gain  Gain=web_psb/L  SaturateOnIntegerOverflow=on
  Integrator3 : Integrator  InitialCondition=io
  R : Gain  Orientation=left  Gain=R  SaturateOnIntegerOverflow=on
  Sum5 : Sum  Inputs=-+-  SaturateOnIntegerOverflow=on  InputSameDT=on
  i : Outport  InitialOutput=0
  wires:
  Integrator3/1 -> i/1, R/1
  1/L/1 -> Integrator3/1
  v/1 -> Sum5/3
  Sum5/1 -> 1/L/1
  R/1 -> Sum5/1
  e/1 -> Sum5/2

== system powerlib_models/Continuous/simplified_sync_mach/gen ==
  note: This subsystem generates the 3 line-to-neutral voltages inside the machine.
  theta : Inport  Port=1  LatchInput=off
  E : Inport  Port=2  LatchInput=off
  Vn : Inport  Port=3  LatchInput=off
  1_Vb2 : Gain  Gain=1/Vb2  SaturateOnIntegerOverflow=on
  Mux : Mux  Inputs=3
  Product : Product  SaturateOnIntegerOverflow=on  InputSameDT=on
  Sum : Sum  Inputs=|++  SaturateOnIntegerOverflow=on  InputSameDT=on
  Sum1 : Sum  Orientation=down  Inputs=--  SaturateOnIntegerOverflow=on  InputSameDT=on
  rem(wt,2pi) : Fcn  Expr=rem(u[1],2*pi)
  sin(a) : Fcn  Expr=sin(u)
  sin(b) : Fcn  Expr=sin(u-pi23)
  e : Outport  InitialOutput=0
  wires:
  rem(wt,2pi)/1 -> sin(a)/1, sin(b)/1
  theta/1 -> rem(wt,2pi)/1
  sin(a)/1 -> Sum1/2, Mux/1
  Sum1/1 -> Mux/3
  sin(b)/1 -> Sum1/1, Mux/2
  E/1 -> 1_Vb2/1
  1_Vb2/1 -> Product/2
  Vn/1 -> Sum/2
  Mux/1 -> Product/1
  Product/1 -> Sum/1
  Sum/1 -> e/1

== system powerlib_models/Continuous/simplified_sync_mach/wattmeter ==
  note: This subsystem computes the total electrical
      | power delivered or absorbed by the machine.
  i : Inport  Port=1  LatchInput=off
  v : Inport  Port=2  LatchInput=off
  2_3 : Gain  Gain=2/3  SaturateOnIntegerOverflow=on
  Product : Product  SaturateOnIntegerOverflow=on  InputSameDT=on
  Sum : Sum  Inputs=+  SaturateOnIntegerOverflow=on  InputSameDT=on
  Pe : Outport  InitialOutput=0
  wires:
  Product/1 -> Sum/1
  i/1 -> Product/1
  v/1 -> Product/2
  Sum/1 -> 2_3/1
  2_3/1 -> Pe/1

== system powerlib_models/Continuous/synchronous_machine/Delta angle ==
  Vq : Inport  Port=1  PortDimensions=1  LatchInput=off
  Vd : Inport  Port=2  PortDimensions=1  LatchInput=off
  Cartesian to Polar : Subsystem
      mask Type: Cart2Polar
      mask Description:
      | Transformation from cartesian to polar coordinates.
      | [x, y] -> [r, theta]
      | 
      | r = sqrt(x^2 + y^2);
      | theta = atan(y/x);
      mask Help: Unmask this block for more help.
      mask Display: plot(0,0,100,100,[24,20,15,20,20],[85,95,85,95,20],[80,20,95,85,95,85],[70,20,20,15,20,24],[56,56,55,52,50,46],[20,26,31,35,38,42])
  Radians to Degrees : Subsystem
      mask Type: RadiansToDegrees
      mask Description:
      | Conversion from Radians to Degrees.
      | 
      | D=180/pi*R
      mask Help: This block converts from Radians to Degrees.
      mask Display: disp('R2D')
  Terminator2 : Terminator
  delta : Outport
  wires:
  Cartesian to Polar/2(theta) -> Radians to Degrees/1(Radians in)
  Cartesian to Polar/1(r) -> Terminator2/1
  Vq/1 -> Cartesian to Polar/1(x)
  Radians to Degrees/1(Degrees out) -> delta/1  "delta"
  Vd/1 -> Cartesian to Polar/2(y)

== system powerlib_models/Continuous/synchronous_machine/PQ ==
  note: PQ Measurement:
  note: Q = Vq*Id-Vd*Iq
  note: P = Vd*Id + Vq*Iq
  Vq : Inport  Port=1  PortDimensions=1  LatchInput=off
  Vd : Inport  Port=2  PortDimensions=1  LatchInput=off
  Iq : Inport  Port=3  PortDimensions=2  LatchInput=off
  Demux1 : Demux  Outputs=[1,1]
  Gain : Gain  Gain=Gain1  SaturateOnIntegerOverflow=on
  Gain1 : Gain  Gain=Gain1  SaturateOnIntegerOverflow=on
  Product{2..5} (4 alike) : Product  SaturateOnIntegerOverflow=on  InputSameDT=on
  Sum : Sum  SaturateOnIntegerOverflow=on  InputSameDT=on
  Sum1 : Sum  Inputs=+-  SaturateOnIntegerOverflow=on  InputSameDT=on
  Peo : Outport
  Qeo : Outport  Port=2
  wires:
  Demux1/2 -> Product4/2, Product3/2
  Vq/1 -> Product4/1, Product2/1
  Vd/1 -> Product5/1, Product3/1
  Sum1/1 -> Gain1/1  "Qeo"
  Sum/1 -> Gain/1  "Peo"
  Product5/1 -> Sum1/2
  Product4/1 -> Sum1/1
  Product3/1 -> Sum/2
  Product2/1 -> Sum/1
  Gain/1 -> Peo/1
  Gain1/1 -> Qeo/1
  Iq/1 -> Demux1/1
  Demux1/1 -> Product2/2, Product5/2

== system powerlib_models/Continuous/synchronous_machine/Subsystem ==
  Vf : Inport  Port=1  PortDimensions=1  LatchInput=off
  Constant : Constant  Value=excAxis
  Ground2 : Ground
  Switch : Switch  Threshold=1.5  InputSameDT=on
  Switch1 : Switch  Threshold=1.5  InputSameDT=on
  Vkq1 : Outport
  Vfd : Outport  Port=2
  wires:
  Ground2/1 -> Switch1/1, Switch/3
  Vf/1 -> Switch1/3, Switch/1
  Constant/1 -> Switch/2, Switch1/2
  Switch1/1 -> Vfd/1
  Switch/1 -> Vkq1/1

== system powerlib_models/Continuous/synchronous_machine/abc2qd ==
  note: This subsystem converts Vab and Vbc to Vd,Vq. The sine and cosine com-
      | puted here are sent to the inverse transformation subsystem qd/abc.
  v : Inport  Port=1  PortDimensions=2  LatchInput=off
  theta : Inport  Port=2  PortDimensions=1  LatchInput=off
  1_Vb : Gain  Gain=1/Vb  SaturateOnIntegerOverflow=on
  Elementary Math : ElementaryMath
  Elementary Math1 : ElementaryMath  Operator=cos
  Fcn2 : Fcn  Expr=(u[4]*(2*u[1]+u[2]) + (sqrt3*u[2]*u[3])) * one_third
  Fcn3 : Fcn  Expr=(u[3]*(2*u[1]+u[2]) + (-sqrt3*u[2]*u[4])) * one_third
  Mux1 : Mux  Inputs=[ 2 2 ]
  Mux3 : Mux  Inputs=2
  cos,sin : Outport  InitialOutput=0
  vq : Outport  Port=2  InitialOutput=0
  vd : Outport  Port=3  InitialOutput=0
  wires:
  1_Vb/1 -> Mux1/1
  v/1 -> 1_Vb/1
  Mux1/1 -> Fcn2/1, Fcn3/1
  Mux3/1 -> Mux1/2, cos,sin/1
  theta/1 -> Elementary Math/1, Elementary Math1/1
  Elementary Math/1 -> Mux3/1
  Elementary Math1/1 -> Mux3/2
  Fcn2/1 -> vq/1  "vq"
  Fcn3/1 -> vd/1  "vd"

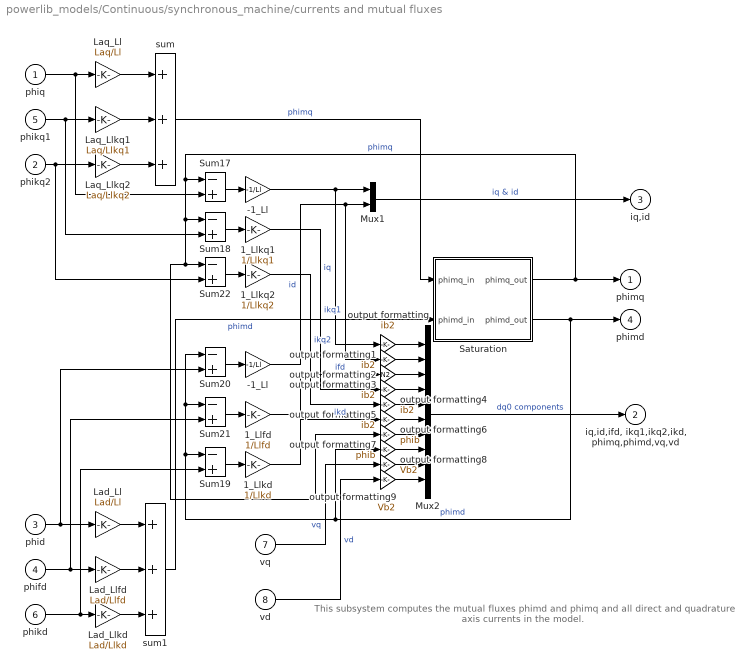
== system powerlib_models/Continuous/synchronous_machine/currents and mutual fluxes ==
  note: This subsystem computes the mutual fluxes phimd
      | and phimq and all direct and quadrature axis
      | currents in the model.
  phiq : Inport  Port=1  PortDimensions=1  LatchInput=off
  phikq2 : Inport  Port=2  PortDimensions=1  LatchInput=off
  phid : Inport  Port=3  PortDimensions=1  LatchInput=off
  phifd : Inport  Port=4  PortDimensions=1  LatchInput=off
  phikq1 : Inport  Port=5  PortDimensions=1  LatchInput=off
  phikd : Inport  Port=6  PortDimensions=1  LatchInput=off
  vq : Inport  Port=7  PortDimensions=1  LatchInput=off
  vd : Inport  Port=8  PortDimensions=1  LatchInput=off
  -1_Ll : Gain  Gain=-1/Ll  SaturateOnIntegerOverflow=on
  "-1_Ll " : Gain  Gain=-1/Ll  SaturateOnIntegerOverflow=on
  1_Llfd : Gain  Gain=1/Llfd  SaturateOnIntegerOverflow=on
  1_Llkd : Gain  Gain=1/Llkd  SaturateOnIntegerOverflow=on
  1_Llkq1 : Gain  Gain=1/Llkq1  SaturateOnIntegerOverflow=on
  1_Llkq2 : Gain  Gain=1/Llkq2  SaturateOnIntegerOverflow=on
  Lad_Ll : Gain  Gain=Lad/Ll  SaturateOnIntegerOverflow=on
  Lad_Llfd : Gain  Gain=Lad/Llfd  SaturateOnIntegerOverflow=on
  Lad_Llkd : Gain  Gain=Lad/Llkd  SaturateOnIntegerOverflow=on
  Laq_Ll : Gain  Gain=Laq/Ll  SaturateOnIntegerOverflow=on
  Laq_Llkq1 : Gain  Gain=Laq/Llkq1  SaturateOnIntegerOverflow=on
  Laq_Llkq2 : Gain  Gain=Laq/Llkq2  SaturateOnIntegerOverflow=on
  Mux1 : Mux  Inputs=2
  Mux2 : Mux  Inputs=[1,1,1,1,1,1,1,1,1,1]
  Saturation : Subsystem
  Sum{17..22} (6 alike) : Sum  Inputs=-+  SaturateOnIntegerOverflow=on  InputSameDT=on
  output formatting{,1,3..5} (5 alike) : Gain  Gain=ib2  SaturateOnIntegerOverflow=on
  output formatting2 : Gain  Gain=N2  SaturateOnIntegerOverflow=on
  output formatting6 : Gain  Gain=phib  SaturateOnIntegerOverflow=on
  output formatting7 : Gain  Gain=phib  SaturateOnIntegerOverflow=on
  output formatting8 : Gain  Gain=Vb2  SaturateOnIntegerOverflow=on
  output formatting9 : Gain  Gain=Vb2  SaturateOnIntegerOverflow=on
  sum : Sum  Inputs=+++  SaturateOnIntegerOverflow=on  InputSameDT=on
  sum1 : Sum  Inputs=+++  SaturateOnIntegerOverflow=on  InputSameDT=on
  phimq : Outport  InitialOutput=0
  "iq,id,ifd, ikq1,ikq2,ikd, phimq,phimd,vq,vd" : Outport  Port=2  InitialOutput=0
  iq,id : Outport  Port=3  InitialOutput=0
  phimd : Outport  Port=4  InitialOutput=0
  wires:
  Saturation/2(phimd_out) -> Sum19/1, Sum21/1, Sum20/1, output formatting7/1, phimd/1  "phimd"
  Saturation/1(phimq_out) -> Sum17/1, Sum22/1, output formatting6/1, Sum18/1, phimq/1  "phimq"
  sum1/1 -> Saturation/2(phimd_in)  "phimd"
  sum/1 -> Saturation/1(phimq_in)  "phimq"
  1_Llkq2/1 -> output formatting4/1  "ikq2"
  1_Llkq1/1 -> output formatting3/1  "ikq1"
  Sum20/1 -> "-1_Ll "/1
  "-1_Ll "/1 -> Mux1/2, output formatting1/1  "id"
  Sum21/1 -> 1_Llfd/1
  Sum19/1 -> 1_Llkd/1
  1_Llfd/1 -> output formatting2/1  "ifd"
  1_Llkd/1 -> output formatting5/1  "ikd"
  Sum18/1 -> 1_Llkq1/1
  Sum17/1 -> -1_Ll/1
  Sum22/1 -> 1_Llkq2/1
  -1_Ll/1 -> Mux1/1, output formatting/1  "iq"
  Mux1/1 -> iq,id/1  "iq & id"
  Lad_Llkd/1 -> sum1/3
  Lad_Llfd/1 -> sum1/2
  Lad_Ll/1 -> sum1/1
  phifd/1 -> Lad_Llfd/1, Sum21/2
  phid/1 -> Sum20/2, Lad_Ll/1
  phikd/1 -> Lad_Llkd/1, Sum19/2
  phiq/1 -> Laq_Ll/1, Sum17/2
  Laq_Ll/1 -> sum/1
  Laq_Llkq2/1 -> sum/3
  Laq_Llkq1/1 -> sum/2
  phikq2/1 -> Laq_Llkq2/1, Sum22/2
  phikq1/1 -> Laq_Llkq1/1, Sum18/2
  vq/1 -> output formatting8/1  "vq"
  vd/1 -> output formatting9/1  "vd"
  Mux2/1 -> "iq,id,ifd, ikq1,ikq2,ikd, phimq,phimd,vq,vd"/1  "dq0 components"
  output formatting/1 -> Mux2/1
  output formatting1/1 -> Mux2/2
  output formatting2/1 -> Mux2/3
  output formatting3/1 -> Mux2/4
  output formatting4/1 -> Mux2/5
  output formatting5/1 -> Mux2/6
  output formatting6/1 -> Mux2/7
  output formatting7/1 -> Mux2/8
  output formatting8/1 -> Mux2/9
  output formatting9/1 -> Mux2/10

== system powerlib_models/Continuous/synchronous_machine/phid ==
  note: This subsystem computes the direct axis flux phid.
  w : Inport  Port=1  PortDimensions=1  LatchInput=off
  phiq : Inport  Port=2  PortDimensions=1  LatchInput=off
  vd : Inport  Port=3  PortDimensions=1  LatchInput=off
  phimd : Inport  Port=4  PortDimensions=1  LatchInput=off
  Product1 : Product  SaturateOnIntegerOverflow=on  InputSameDT=on
  Rs_Ll : Gain  Gain=Rs/Ll  SaturateOnIntegerOverflow=on
  Sum2 : Sum  Inputs=+++  SaturateOnIntegerOverflow=on  InputSameDT=on
  Sum9 : Sum  Inputs=+-  SaturateOnIntegerOverflow=on  InputSameDT=on
  int : Integrator  InitialCondition=phido
  web_psb : Gain  Gain=web_psb  SaturateOnIntegerOverflow=on
  phid : Outport  InitialOutput=0
  wires:
  phimd/1 -> Sum9/1
  vd/1 -> Sum2/2
  phiq/1 -> Product1/2
  w/1 -> Product1/1
  Product1/1 -> Sum2/1
  Sum9/1 -> Rs_Ll/1
  Rs_Ll/1 -> Sum2/3
  Sum2/1 -> web_psb/1
  web_psb/1 -> int/1
  int/1 -> phid/1, Sum9/2

== system powerlib_models/Continuous/synchronous_machine/phifd ==
  note: This subsystem computes the field flux phifd.
  vfd : Inport  Port=1  PortDimensions=1  LatchInput=off
  phimd : Inport  Port=2  PortDimensions=1  LatchInput=off
  N : Gain  Gain=N  SaturateOnIntegerOverflow=on
  Rf_Llfd : Gain  Gain=Rf/Llfd  SaturateOnIntegerOverflow=on
  Sum10 : Sum  Inputs=+-  SaturateOnIntegerOverflow=on  InputSameDT=on
  Sum3 : Sum  SaturateOnIntegerOverflow=on  InputSameDT=on
  int : Integrator  InitialCondition=phifdo
  web_psb : Gain  Gain=web_psb  SaturateOnIntegerOverflow=on
  phifd : Outport  InitialOutput=0
  wires:
  N/1 -> Sum3/1
  vfd/1 -> N/1
  Rf_Llfd/1 -> Sum3/2
  Sum10/1 -> Rf_Llfd/1
  phimd/1 -> Sum10/1
  web_psb/1 -> int/1
  int/1 -> phifd/1, Sum10/2
  Sum3/1 -> web_psb/1

== system powerlib_models/Continuous/synchronous_machine/phikd ==
  note: This subsystem computes the direct axis damper flux phikd.
  phimd : Inport  Port=1  PortDimensions=1  LatchInput=off
  vkd : Inport  Port=2  PortDimensions=1  LatchInput=off
  Rkd_Llkd : Gain  Gain=Rkd/Llkd  SaturateOnIntegerOverflow=on
  Sum11 : Sum  Inputs=-+  SaturateOnIntegerOverflow=on  InputSameDT=on
  Sum4 : Sum  SaturateOnIntegerOverflow=on  InputSameDT=on
  int : Integrator  InitialCondition=phikdo
  web_psb : Gain  Gain=web_psb  SaturateOnIntegerOverflow=on
  phikd : Outport  InitialOutput=0
  wires:
  Rkd_Llkd/1 -> Sum4/1
  Sum11/1 -> Rkd_Llkd/1
  phimd/1 -> Sum11/2
  vkd/1 -> Sum4/2
  web_psb/1 -> int/1
  int/1 -> phikd/1, Sum11/1
  Sum4/1 -> web_psb/1

== system powerlib_models/Continuous/synchronous_machine/phikq1 ==
  note: This subsystem computes the quadrature axis damper flux phikq.
  phimq : Inport  Port=1  PortDimensions=1  LatchInput=off
  vkq1 : Inport  Port=2  PortDimensions=1  LatchInput=off
  Rkq1_Llkq1 : Gain  Gain=Rkq1/Llkq1  SaturateOnIntegerOverflow=on
  Sum1 : Sum  SaturateOnIntegerOverflow=on  InputSameDT=on
  Sum7 : Sum  Inputs=-+  SaturateOnIntegerOverflow=on  InputSameDT=on
  int : Integrator  InitialCondition=phikq1o
  web_psb : Gain  Gain=web_psb  SaturateOnIntegerOverflow=on
  phikq1 : Outport  InitialOutput=0
  wires:
  int/1 -> Sum7/1, phikq1/1
  web_psb/1 -> int/1
  vkq1/1 -> Sum1/2
  phimq/1 -> Sum7/2
  Sum1/1 -> web_psb/1
  Sum7/1 -> Rkq1_Llkq1/1
  Rkq1_Llkq1/1 -> Sum1/1

== system powerlib_models/Continuous/synchronous_machine/phikq2 ==
  note: This subsystem computes the quadrature axis damper flux phikq2.
  vkq2 : Inport  Port=1  PortDimensions=1  LatchInput=off
  phimq : Inport  Port=2  PortDimensions=1  LatchInput=off
  Enabled integrator : Subsystem  TreatAsAtomicUnit=on
      mask Display: disp('1/s')
  Rkq2_Llkq2 : Gain  Gain=Rkq2/Llkq2  SaturateOnIntegerOverflow=on
  Sum1 : Sum  SaturateOnIntegerOverflow=on  InputSameDT=on
  Sum7 : Sum  Inputs=-+  SaturateOnIntegerOverflow=on  InputSameDT=on
  web_psb : Gain  Gain=web_psb  SaturateOnIntegerOverflow=on
  wref : Constant  Value=isfinite(Llkq2)
  phikq2 : Outport  InitialOutput=0
  wires:
  wref/1 -> Enabled integrator/Enable
  Enabled integrator/1(Out1) -> phikq2/1, Sum7/1
  web_psb/1 -> Enabled integrator/1(In1)
  Sum7/1 -> Rkq2_Llkq2/1
  vkq2/1 -> Sum1/2
  Rkq2_Llkq2/1 -> Sum1/1
  Sum1/1 -> web_psb/1
  phimq/1 -> Sum7/2

== system powerlib_models/Continuous/synchronous_machine/phiq ==
  note: This subsystem computes the quadrature axis flux phiq.
  vq : Inport  Port=1  PortDimensions=1  LatchInput=off
  w : Inport  Port=2  PortDimensions=1  LatchInput=off
  phid : Inport  Port=3  PortDimensions=1  LatchInput=off
  phimq : Inport  Port=4  PortDimensions=1  LatchInput=off
  Product2 : Product  SaturateOnIntegerOverflow=on  InputSameDT=on
  Rs_Ll : Gain  Gain=Rs/Ll  SaturateOnIntegerOverflow=on
  Sum : Sum  Inputs=+-+  SaturateOnIntegerOverflow=on  InputSameDT=on
  Sum6 : Sum  Inputs=+-  SaturateOnIntegerOverflow=on  InputSameDT=on
  int1 : Integrator  InitialCondition=phiqo
  web_psb : Gain  Gain=web_psb  SaturateOnIntegerOverflow=on
  phiq : Outport  InitialOutput=0
  wires:
  Sum/1 -> web_psb/1
  Rs_Ll/1 -> Sum/3
  Sum6/1 -> Rs_Ll/1
  Product2/1 -> Sum/2
  vq/1 -> Sum/1
  w/1 -> Product2/1
  phid/1 -> Product2/2
  phimq/1 -> Sum6/1
  web_psb/1 -> int1/1
  int1/1 -> phiq/1, Sum6/2

== system powerlib_models/Continuous/synchronous_machine/qd2abc ==
  note: This subsystem converts id,iq to ia,ib,ic.
  sin,cos : Inport  Port=1  PortDimensions=2  LatchInput=off
  iq,id : Inport  Port=2  PortDimensions=2  LatchInput=off
  Fcn : Fcn  Expr=u[3]*u[2] + u[4]*u[1]
  Fcn1 : Fcn  Expr=(u[2]*(-u[3]-sqrt3*u[4]) + u[1]*(sqrt3*u[3]-u[4]))*0.5
  Mux : Mux  Inputs=[ 2 2 ]
  Mux1 : Mux  Inputs=[1,1,1]
  Mux1_ : Mux  Inputs=3
  Sum : Sum  Orientation=down  Inputs=--  SaturateOnIntegerOverflow=on  InputSameDT=on
  ib : Gain  Gain=ib  SaturateOnIntegerOverflow=on
  output formatting : Gain  Gain=ib2  SaturateOnIntegerOverflow=on
  output formatting1 : Gain  Gain=ib2  SaturateOnIntegerOverflow=on
  output formatting2 : Gain  Gain=ib2  SaturateOnIntegerOverflow=on
  is(A) : Outport  InitialOutput=0
  is(pu) : Outport  Port=2  InitialOutput=0
  wires:
  iq,id/1 -> Mux/2
  sin,cos/1 -> Mux/1
  Mux/1 -> Fcn1/1, Fcn/1
  Mux1_/1 -> ib/1
  Sum/1 -> Mux1_/3, output formatting2/1  "is_c"
  Fcn/1 -> Sum/1, Mux1_/1, output formatting/1  "is_a"
  Fcn1/1 -> Sum/2, Mux1_/2, output formatting1/1  "is_b"
  ib/1 -> is(A)/1
  Mux1/1 -> is(pu)/1  "Stator currents"
  output formatting/1 -> Mux1/1  "is_a"
  output formatting1/1 -> Mux1/2  "is_b"
  output formatting2/1 -> Mux1/3  "is_c"

== system powerlib_models/Continuous/thyristor (logical)/Break Alg. Loop ==
  In1 : Inport  Port=1  LatchInput=off
  0 2 : Constant  Value=0.001
  Data Type  Conversion : DataTypeConversion  OutDataTypeMode=double  SaturateOnIntegerOverflow=on  RndMeth=Zero
  Data Type  Conversion1 : DataTypeConversion  OutDataTypeMode=double  SaturateOnIntegerOverflow=on  RndMeth=Zero
  Integrator : Integrator  LimitOutput=on  UpperSaturationLimit=0.00101
  R_device : Gain  Gain=1e7  SaturateOnIntegerOverflow=on
  Relational Operator1 : RelationalOperator  Operator=>  InputSameDT=on
  Vak-Vf-Ron*Iak : Sum  Inputs=+-  SaturateOnIntegerOverflow=on  InputSameDT=on
  Out1 : Outport
  wires:
  Relational Operator1/1 -> Data Type  Conversion/1
  0 2/1 -> Relational Operator1/2
  Integrator/1 -> Relational Operator1/1, Vak-Vf-Ron*Iak/2
  Vak-Vf-Ron*Iak/1 -> R_device/1
  R_device/1 -> Integrator/1
  Data Type  Conversion1/1 -> Vak-Vf-Ron*Iak/1
  In1/1 -> Data Type  Conversion1/1
  Data Type  Conversion/1 -> Out1/1
